simulink model "HVAC"  (R2020a)
settings: Solver=VariableStepAuto  StartTime=0.0  StopTime=1740  RelTol=1e-3
values from neighbouring files (symbols this model uses):
  A_dor = 1.85    [Parameter.m]
  beta_pas = 1.8    [Parameter.m]
  c_p = 1.005    [Parameter.m]
  Ca = 0.1    [Parameter.m]
  m_air = 111    [Parameter.m]
  phi_vnt = 0.2    [Parameter.m]
  pho_air = 1.2258    [Parameter.m]
  R_p = 0.3    [Parameter.m]
  T_set = 20    [Parameter.m]
  T_umgebung = 5    [Parameter.m]
  V_hvac = 1.13    [Parameter.m]
libraries: simulink x1
settings Model: Creator=zf  LastModifiedBy=zf

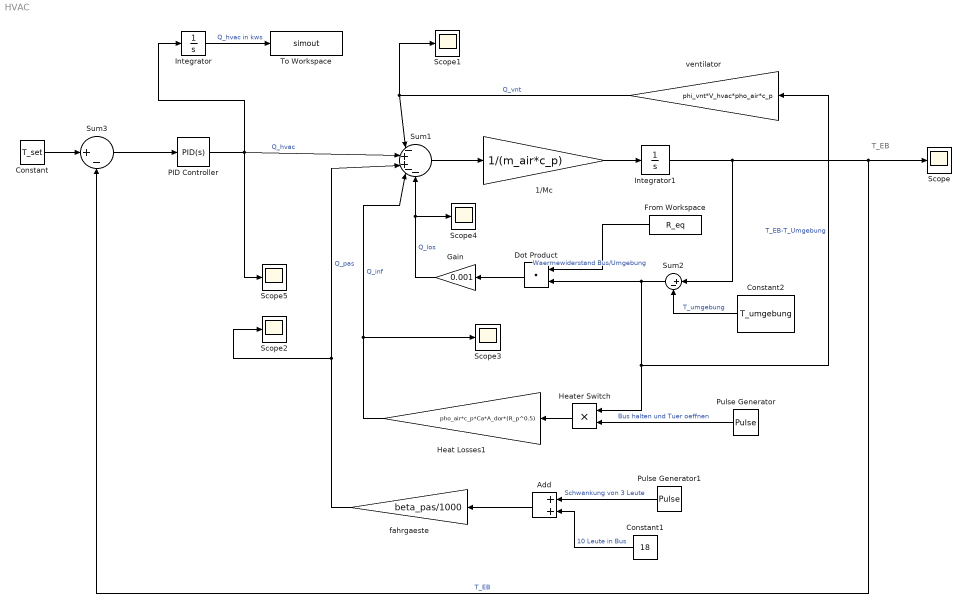
== system HVAC ==
  note: T_EB
  1/Mc : Gain  Gain=1/(m_air*c_p)  SaturateOnIntegerOverflow=on  OutDataTypeStr=Inherit: Same as input  ParamDataTypeStr=Inherit: Same as input
  Add : Sum
  Constant : Constant  Value=T_set
  Constant1 : Constant  Value=18
  Constant2 : Constant  Value=T_umgebung
  Dot Product : DotProduct  InputSameDT=on  OutDataTypeStr=Inherit: Inherit via internal rule
  From Workspace : FromWorkspace  VariableName=R_eq
  Gain : Gain  Gain=0.001
  Heat Losses1 : Gain  Gain=pho_air*c_p*Ca*A_dor*(R_p^0.5)  SaturateOnIntegerOverflow=on  OutDataTypeStr=Inherit: Same as input  ParamDataTypeStr=Inherit: Same as input
  Heater Switch : Product  RndMeth=Zero
  Integrator : Integrator
  Integrator1 : Integrator  InitialCondition=20
  PID Controller : simulink/Continuous/PID Controller  Controller=PID  Form=Parallel  TimeDomain=Continuous-time  UseExternalTs=off  SampleTime=-1  IntegratorMethod=Forward Euler  FilterMethod=Forward Euler  ControllerParametersSource=internal  P=77.1066651185351  I=79.939420918431  D=-7.83735729640915  UseFilter=on  N=9.83835012266993  TunerSelectOption=Transfer Function Based (PID Tuner App)  InitialConditionSource=internal  InitialConditionForIntegrator=0  InitialConditionForFilter=0  DifferentiatorICPrevScaledInput=0  ExternalReset=none  TrackingMode=off  Kt=1  LimitOutput=off  UpperSaturationLimit=inf  LowerSaturationLimit=-inf  LinearizeAsGain=on  AntiWindupMode=none  Kb=1  POutMin=[]  POutMax=[]  IOutMin=[]  IOutMax=[]  DOutMin=[]  DOutMax=[]  NOutMin=[]  NOutMax=[]  SumOutMin=[]  SumOutMax=[]  SaturationOutMin=[]  SaturationOutMax=[]  PParamMin=[]  PParamMax=[]  IParamMin=[]  IParamMax=[]  DParamMin=[]  DParamMax=[]  NParamMin=[]  NParamMax=[]  KbParamMin=[]  KbParamMax=[]  KtParamMin=[]  KtParamMax=[]  KbOutMin=[]  KbOutMax=[]  KtOutMin=[]  KtOutMax=[]  IntegratorOutMin=[]  IntegratorOutMax=[]  FilterOutMin=[]  FilterOutMax=[]  SumI1OutMin=[]  SumI1OutMax=[]  SumI2OutMin=[]  SumI2OutMax=[]  SumI3OutMin=[]  SumI3OutMax=[]  SumI4OutMin=[]  SumI4OutMax=[]  SumDOutMin=[]  SumDOutMax=[]  DifferentiatorOutMin=[]  DifferentiatorOutMax=[]  FilterDiffOutCoefMin=[]  FilterDiffOutCoefMax=[]  ReciprocalOutMin=[]  ReciprocalOutMax=[]  SumDenOutMin=[]  SumDenOutMax=[]  SumNumOutMin=[]  SumNumOutMax=[]  DivideOutMin=[]  DivideOutMax=[]  UdiffTsProdOutMin=[]  UdiffTsProdOutMax=[]  NTsProdOutMin=[]  NTsProdOutMax=[]  UintegralTsProdOutMin=[]  UintegralTsProdOutMax=[]  UngainTsProdOutMin=[]  UngainTsProdOutMax=[]  IntegratorContinuousStateAttributes=''  IntegratorStateMustResolveToSignalObject=off  IntegratorRTWStateStorageClass=Auto  FilterContinuousStateAttributes=''  FilterStateMustResolveToSignalObject=off  FilterRTWStateStorageClass=Auto  ParallelPVariant=InternalParameters  IdealPVariant=Disabled  IVariant=InternalParameters  DVariant=InternalParameters  IntegratorVariant=Continuous  SatVariant=Disabled  AWVariant=Passthrough  PCopyVariant=Disabled  TRVariant=Disabled  FdbkBlocksVariant=Forward  IdealPFdbkVariant=Disabled  SatFdbkVariant=Disabled  DerivativeFilterVariant=ContFilter  NVariant=InternalParameters  NCopyVariant=Disabled  FilterICVariant=InternalICsFilter  IntegratorICVariant=InternalICs  ExternalResetVariant=Disabled  TRSumVariant=Passthrough  SumFdbkVariant=Disabled  SumVariant=Sum_PID  TsampFilterVariant=InternalTs  TsampNgainVariant=Passthrough  TsampIntegralVariant=Passthrough
  Pulse Generator : DiscretePulseGenerator  PulseType=Time based  Period=150  PulseWidth=20
  Pulse Generator1 : DiscretePulseGenerator  PulseType=Time based  Amplitude=5.4  Period=240  PulseWidth=50
  Scope{,1..5} (6 alike) : Scope
  Sum1 : Sum  Inputs=|-++--  InputSameDT=on  SaturateOnIntegerOverflow=on  OutDataTypeStr=Inherit: Same as first input
  Sum2 : Sum  Inputs=|+-  InputSameDT=on  SaturateOnIntegerOverflow=on  OutDataTypeStr=Inherit: Same as first input
  Sum3 : Sum  Inputs=|+-  InputSameDT=on  SaturateOnIntegerOverflow=on  OutDataTypeStr=Inherit: Same as first input
  To Workspace : ToWorkspace  VariableName=simout  SaveFormat=Timeseries  SampleTime=-1
  fahrgaeste : Gain  Gain=beta_pas/1000  SaturateOnIntegerOverflow=on  OutDataTypeStr=Inherit: Same as input  ParamDataTypeStr=Inherit: Same as input
  ventilator : Gain  Gain=phi_vnt*V_hvac*pho_air*c_p  SaturateOnIntegerOverflow=on  OutDataTypeStr=Inherit: Same as input  ParamDataTypeStr=Inherit: Same as input
  wires:
  1/Mc/1 -> Integrator1/1
  Integrator1/1 -> Scope/1, Sum3/2, Sum2/1  "T_EB"
  Constant2/1 -> Sum2/2  "T_umgebung"
  Sum2/1 -> Dot Product/2, Heater Switch/1, ventilator/1  "T_EB-T_Umgebung"
  Dot Product/1 -> Gain/1
  Sum1/1 -> 1/Mc/1
  ventilator/1 -> Scope1/1, Sum1/1  "Q_vnt"
  Pulse Generator/1 -> Heater Switch/2  "Bus halten und Tuer oeffnen"
  Heater Switch/1 -> Heat Losses1/1
  Heat Losses1/1 -> Sum1/4, Scope3/1  "Q_inf"
  fahrgaeste/1 -> Sum1/3, Scope2/1  "Q_pas"
  Pulse Generator1/1 -> Add/1  "Schwankung von 3 Leute"
  Constant/1 -> Sum3/1
  Sum3/1 -> PID Controller/1
  Constant1/1 -> Add/2  "10 Leute in Bus"
  Add/1 -> fahrgaeste/1
  From Workspace/1 -> Dot Product/1  "Waermewiderstand Bus/Umgebung"
  Gain/1 -> Sum1/5, Scope4/1  "Q_los"
  PID Controller/1 -> Sum1/2, Integrator/1, Scope5/1  "Q_hvac"
  Integrator/1 -> To Workspace/1  "Q_hvac in kws"
